simulink model "TST_OilP_DD"  (R2016b)
settings: Solver=FixedStepDiscrete  StartTime=0.0  StopTime=simTime  FixedStep=sampleTime  RelTol=1e-3
values from neighbouring files (symbols this model uses):
  testCase = 1    [initTST_OilP_DD_001.m]
libraries: simulink x13, UnitTest_Lib x11
settings Model: Creator=xinchangran  LastModifiedBy=xinchangran
settings DebuggingCC: SignalRangeChecking=error

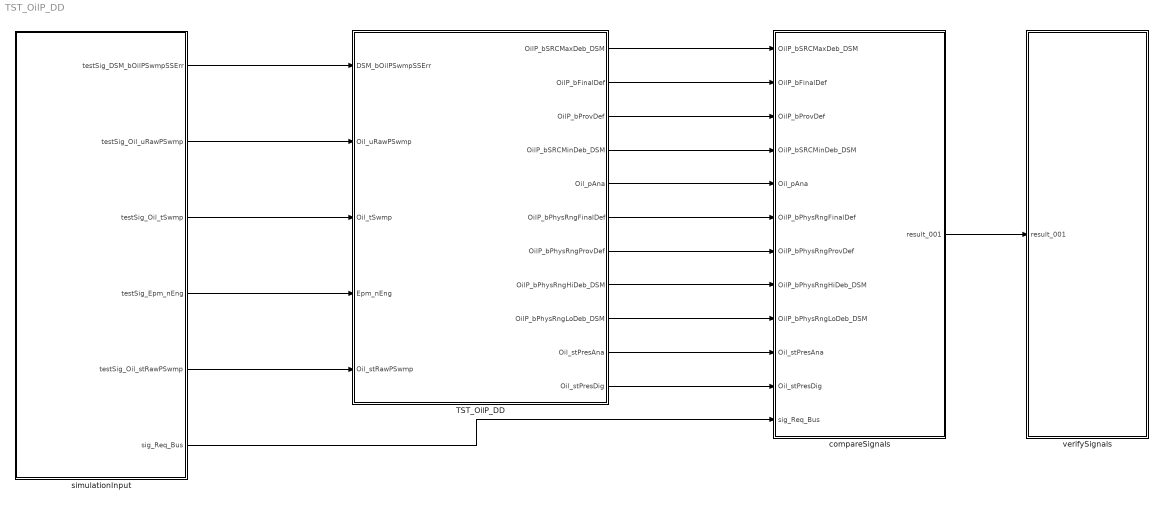
== system TST_OilP_DD ==
  TST_OilP_DD : Subsystem
  compareSignals : Subsystem
  simulationInput : Subsystem
  verifySignals : Subsystem
  wires:
  simulationInput/1(testSig_DSM_bOilPSwmpSSErr) -> TST_OilP_DD/1(DSM_bOilPSwmpSSErr)
  simulationInput/2(testSig_Oil_uRawPSwmp) -> TST_OilP_DD/2(Oil_uRawPSwmp)
  simulationInput/3(testSig_Oil_tSwmp) -> TST_OilP_DD/3(Oil_tSwmp)
  simulationInput/4(testSig_Epm_nEng) -> TST_OilP_DD/4(Epm_nEng)
  simulationInput/5(testSig_Oil_stRawPSwmp) -> TST_OilP_DD/5(Oil_stRawPSwmp)
  TST_OilP_DD/1(OilP_bSRCMaxDeb_DSM) -> compareSignals/1(OilP_bSRCMaxDeb_DSM)
  TST_OilP_DD/2(OilP_bFinalDef) -> compareSignals/2(OilP_bFinalDef)
  TST_OilP_DD/3(OilP_bProvDef) -> compareSignals/3(OilP_bProvDef)
  TST_OilP_DD/4(OilP_bSRCMinDeb_DSM) -> compareSignals/4(OilP_bSRCMinDeb_DSM)
  TST_OilP_DD/5(Oil_pAna) -> compareSignals/5(Oil_pAna)
  TST_OilP_DD/6(OilP_bPhysRngFinalDef) -> compareSignals/6(OilP_bPhysRngFinalDef)
  TST_OilP_DD/7(OilP_bPhysRngProvDef) -> compareSignals/7(OilP_bPhysRngProvDef)
  TST_OilP_DD/8(OilP_bPhysRngHiDeb_DSM) -> compareSignals/8(OilP_bPhysRngHiDeb_DSM)
  TST_OilP_DD/9(OilP_bPhysRngLoDeb_DSM) -> compareSignals/9(OilP_bPhysRngLoDeb_DSM)
  TST_OilP_DD/10(Oil_stPresAna) -> compareSignals/10(Oil_stPresAna)
  TST_OilP_DD/11(Oil_stPresDig) -> compareSignals/11(Oil_stPresDig)
  simulationInput/6(sig_Req_Bus) -> compareSignals/12(sig_Req_Bus)
  compareSignals/1(result_001) -> verifySignals/1(result_001)

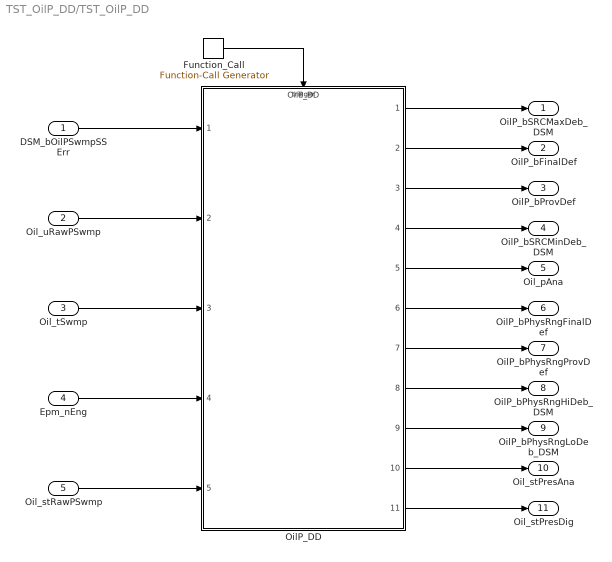
== system TST_OilP_DD/TST_OilP_DD ==
  DSM_bOilPSwmpSSErr : Inport
  Oil_uRawPSwmp : Inport  Port=2
  Oil_tSwmp : Inport  Port=3
  Epm_nEng : Inport  Port=4
  Oil_stRawPSwmp : Inport  Port=5
  Function_Call : simulink/Ports & Subsystems/Function-Call Generator  sample_time=sampleTime  numberOfIterations=1
  OilP_DD : ModelReference  ModelNameDialog=OilP_DD  SimulationMode=Normal  ModelReferenceVersion=1.40  TriggerPortName=function  TriggerPortTriggerType=function-call  TriggerPortStatesWhenEnabling=held
  OilP_bSRCMaxDeb_DSM : Outport
  OilP_bFinalDef : Outport  Port=2
  OilP_bProvDef : Outport  Port=3
  OilP_bSRCMinDeb_DSM : Outport  Port=4
  Oil_pAna : Outport  Port=5
  OilP_bPhysRngFinalDef : Outport  Port=6
  OilP_bPhysRngProvDef : Outport  Port=7
  OilP_bPhysRngHiDeb_DSM : Outport  Port=8
  OilP_bPhysRngLoDeb_DSM : Outport  Port=9
  Oil_stPresAna : Outport  Port=10
  Oil_stPresDig : Outport  Port=11
  wires:
  Function_Call/1 -> OilP_DD/Trigger
  DSM_bOilPSwmpSSErr/1 -> OilP_DD/1
  Oil_uRawPSwmp/1 -> OilP_DD/2
  Oil_tSwmp/1 -> OilP_DD/3
  Epm_nEng/1 -> OilP_DD/4
  Oil_stRawPSwmp/1 -> OilP_DD/5
  OilP_DD/1 -> OilP_bSRCMaxDeb_DSM/1
  OilP_DD/2 -> OilP_bFinalDef/1
  OilP_DD/3 -> OilP_bProvDef/1
  OilP_DD/4 -> OilP_bSRCMinDeb_DSM/1
  OilP_DD/5 -> Oil_pAna/1
  OilP_DD/6 -> OilP_bPhysRngFinalDef/1
  OilP_DD/7 -> OilP_bPhysRngProvDef/1
  OilP_DD/8 -> OilP_bPhysRngHiDeb_DSM/1
  OilP_DD/9 -> OilP_bPhysRngLoDeb_DSM/1
  OilP_DD/10 -> Oil_stPresAna/1
  OilP_DD/11 -> Oil_stPresDig/1

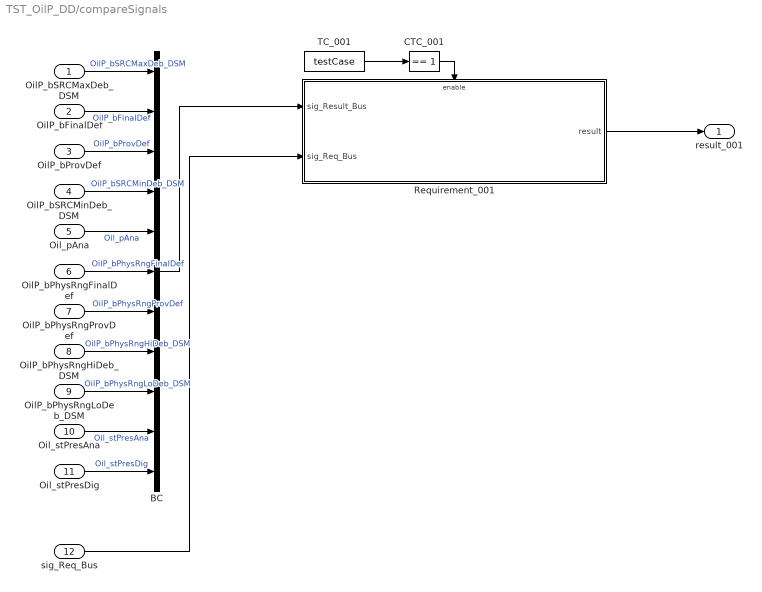
== system TST_OilP_DD/compareSignals ==
  OilP_bSRCMaxDeb_DSM : Inport
  OilP_bFinalDef : Inport  Port=2
  OilP_bProvDef : Inport  Port=3
  OilP_bSRCMinDeb_DSM : Inport  Port=4
  Oil_pAna : Inport  Port=5
  OilP_bPhysRngFinalDef : Inport  Port=6
  OilP_bPhysRngProvDef : Inport  Port=7
  OilP_bPhysRngHiDeb_DSM : Inport  Port=8
  OilP_bPhysRngLoDeb_DSM : Inport  Port=9
  Oil_stPresAna : Inport  Port=10
  Oil_stPresDig : Inport  Port=11
  sig_Req_Bus : Inport  Port=12
  BC : BusCreator  Inputs=11
  CTC_001 : simulink/Logic and Bit Operations/Compare To Constant  relop===  const=1  OutDataTypeStr=boolean
  Requirement_001 : Subsystem
  TC_001 : Constant  Value=testCase
  result_001 : Outport
  wires:
  OilP_bSRCMaxDeb_DSM/1 -> BC/1  "OilP_bSRCMaxDeb_DSM"
  OilP_bFinalDef/1 -> BC/2  "OilP_bFinalDef"
  OilP_bProvDef/1 -> BC/3  "OilP_bProvDef"
  OilP_bSRCMinDeb_DSM/1 -> BC/4  "OilP_bSRCMinDeb_DSM"
  Oil_pAna/1 -> BC/5  "Oil_pAna"
  OilP_bPhysRngFinalDef/1 -> BC/6  "OilP_bPhysRngFinalDef"
  OilP_bPhysRngProvDef/1 -> BC/7  "OilP_bPhysRngProvDef"
  OilP_bPhysRngHiDeb_DSM/1 -> BC/8  "OilP_bPhysRngHiDeb_DSM"
  OilP_bPhysRngLoDeb_DSM/1 -> BC/9  "OilP_bPhysRngLoDeb_DSM"
  Oil_stPresAna/1 -> BC/10  "Oil_stPresAna"
  Oil_stPresDig/1 -> BC/11  "Oil_stPresDig"
  TC_001/1 -> CTC_001/1
  CTC_001/1 -> Requirement_001/Enable
  sig_Req_Bus/1 -> Requirement_001/2(sig_Req_Bus)
  BC/1 -> Requirement_001/1(sig_Result_Bus)
  Requirement_001/1(result) -> result_001/1

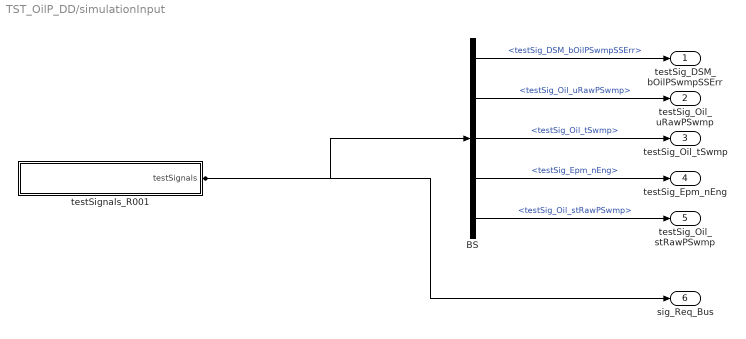
== system TST_OilP_DD/simulationInput ==
  BS : BusSelector  OutputSignals=testSig_DSM_bOilPSwmpSSErr,testSig_Oil_uRawPSwmp,testSig_Oil_tSwmp,testSig_Epm_nEng,testSig_Oil_stRawPSwmp
  testSignals_R001 : Subsystem
  testSig_DSM_bOilPSwmpSSErr : Outport
  testSig_Oil_uRawPSwmp : Outport  Port=2
  testSig_Oil_tSwmp : Outport  Port=3
  testSig_Epm_nEng : Outport  Port=4
  testSig_Oil_stRawPSwmp : Outport  Port=5
  sig_Req_Bus : Outport  Port=6
  wires:
  BS/1 -> testSig_DSM_bOilPSwmpSSErr/1  "<testSig_DSM_bOilPSwmpSSErr>"
  BS/2 -> testSig_Oil_uRawPSwmp/1  "<testSig_Oil_uRawPSwmp>"
  BS/3 -> testSig_Oil_tSwmp/1  "<testSig_Oil_tSwmp>"
  BS/4 -> testSig_Epm_nEng/1  "<testSig_Epm_nEng>"
  BS/5 -> testSig_Oil_stRawPSwmp/1  "<testSig_Oil_stRawPSwmp>"
  testSignals_R001/1(testSignals) -> BS/1, sig_Req_Bus/1

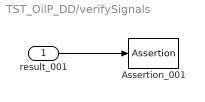
== system TST_OilP_DD/verifySignals ==
  result_001 : Inport
  Assertion_001 : Assertion  Enabled=off
  wires:
  result_001/1 -> Assertion_001/1

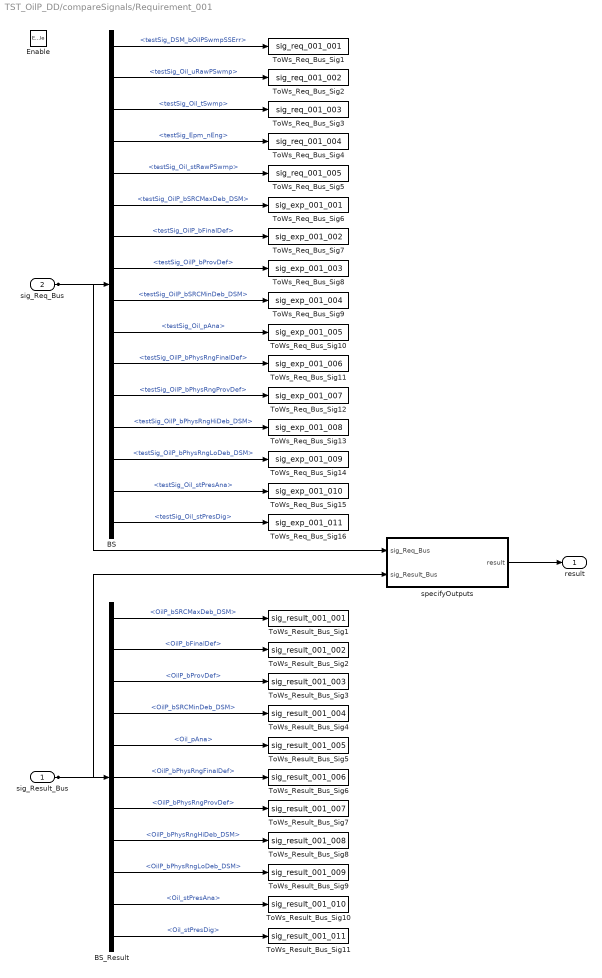
== system TST_OilP_DD/compareSignals/Requirement_001 ==
  sig_Result_Bus : Inport
  sig_Req_Bus : Inport  Port=2
  Enable : EnablePort
  BS : BusSelector  OutputSignals=testSig_DSM_bOilPSwmpSSErr,testSig_Oil_uRawPSwmp,testSig_Oil_tSwmp,testSig_Epm_nEng,testSig_Oil_stRawPSwmp,testSig_OilP_bSRCMaxDeb_DSM,testSig_OilP_bFinalDef,testSig_OilP_bProvDef,testSig_OilP_bSRCMinDeb_DSM,testSig_Oil_pAna,testSig_OilP_bPhysRngFinalDef,testSig_OilP_bPhysRngProvDef,testSig_OilP_bPhysRngHiDeb_DSM,testSig_OilP_bPhysRngLoDeb_DSM,testSig_Oil_stPresAna,testSig_Oil_stPresDig
  BS_Result : BusSelector  OutputSignals=OilP_bSRCMaxDeb_DSM,OilP_bFinalDef,OilP_bProvDef,OilP_bSRCMinDeb_DSM,Oil_pAna,OilP_bPhysRngFinalDef,OilP_bPhysRngProvDef,OilP_bPhysRngHiDeb_DSM,OilP_bPhysRngLoDeb_DSM,Oil_stPresAna,Oil_stPresDig
  ToWs_Req_Bus_Sig1 : ToWorkspace  VariableName=sig_req_001_001  SaveFormat=Structure With Time
  ToWs_Req_Bus_Sig10 : ToWorkspace  VariableName=sig_exp_001_005  SaveFormat=Structure With Time
  ToWs_Req_Bus_Sig11 : ToWorkspace  VariableName=sig_exp_001_006  SaveFormat=Structure With Time
  ToWs_Req_Bus_Sig12 : ToWorkspace  VariableName=sig_exp_001_007  SaveFormat=Structure With Time
  ToWs_Req_Bus_Sig13 : ToWorkspace  VariableName=sig_exp_001_008  SaveFormat=Structure With Time
  ToWs_Req_Bus_Sig14 : ToWorkspace  VariableName=sig_exp_001_009  SaveFormat=Structure With Time
  ToWs_Req_Bus_Sig15 : ToWorkspace  VariableName=sig_exp_001_010  SaveFormat=Structure With Time
  ToWs_Req_Bus_Sig16 : ToWorkspace  VariableName=sig_exp_001_011  SaveFormat=Structure With Time
  ToWs_Req_Bus_Sig2 : ToWorkspace  VariableName=sig_req_001_002  SaveFormat=Structure With Time
  ToWs_Req_Bus_Sig3 : ToWorkspace  VariableName=sig_req_001_003  SaveFormat=Structure With Time
  ToWs_Req_Bus_Sig4 : ToWorkspace  VariableName=sig_req_001_004  SaveFormat=Structure With Time
  ToWs_Req_Bus_Sig5 : ToWorkspace  VariableName=sig_req_001_005  SaveFormat=Structure With Time
  ToWs_Req_Bus_Sig6 : ToWorkspace  VariableName=sig_exp_001_001  SaveFormat=Structure With Time
  ToWs_Req_Bus_Sig7 : ToWorkspace  VariableName=sig_exp_001_002  SaveFormat=Structure With Time
  ToWs_Req_Bus_Sig8 : ToWorkspace  VariableName=sig_exp_001_003  SaveFormat=Structure With Time
  ToWs_Req_Bus_Sig9 : ToWorkspace  VariableName=sig_exp_001_004  SaveFormat=Structure With Time
  ToWs_Result_Bus_Sig1 : ToWorkspace  VariableName=sig_result_001_001  SaveFormat=Structure With Time
  ToWs_Result_Bus_Sig10 : ToWorkspace  VariableName=sig_result_001_010  SaveFormat=Structure With Time
  ToWs_Result_Bus_Sig11 : ToWorkspace  VariableName=sig_result_001_011  SaveFormat=Structure With Time
  ToWs_Result_Bus_Sig2 : ToWorkspace  VariableName=sig_result_001_002  SaveFormat=Structure With Time
  ToWs_Result_Bus_Sig3 : ToWorkspace  VariableName=sig_result_001_003  SaveFormat=Structure With Time
  ToWs_Result_Bus_Sig4 : ToWorkspace  VariableName=sig_result_001_004  SaveFormat=Structure With Time
  ToWs_Result_Bus_Sig5 : ToWorkspace  VariableName=sig_result_001_005  SaveFormat=Structure With Time
  ToWs_Result_Bus_Sig6 : ToWorkspace  VariableName=sig_result_001_006  SaveFormat=Structure With Time
  ToWs_Result_Bus_Sig7 : ToWorkspace  VariableName=sig_result_001_007  SaveFormat=Structure With Time
  ToWs_Result_Bus_Sig8 : ToWorkspace  VariableName=sig_result_001_008  SaveFormat=Structure With Time
  ToWs_Result_Bus_Sig9 : ToWorkspace  VariableName=sig_result_001_009  SaveFormat=Structure With Time
  specifyOutputs : Subsystem
  result : Outport
  wires:
  sig_Req_Bus/1 -> BS/1, specifyOutputs/1(sig_Req_Bus)
  BS/1 -> ToWs_Req_Bus_Sig1/1  "<testSig_DSM_bOilPSwmpSSErr>"
  BS/2 -> ToWs_Req_Bus_Sig2/1  "<testSig_Oil_uRawPSwmp>"
  BS/3 -> ToWs_Req_Bus_Sig3/1  "<testSig_Oil_tSwmp>"
  BS/4 -> ToWs_Req_Bus_Sig4/1  "<testSig_Epm_nEng>"
  BS/5 -> ToWs_Req_Bus_Sig5/1  "<testSig_Oil_stRawPSwmp>"
  BS/6 -> ToWs_Req_Bus_Sig6/1  "<testSig_OilP_bSRCMaxDeb_DSM>"
  BS/7 -> ToWs_Req_Bus_Sig7/1  "<testSig_OilP_bFinalDef>"
  BS/8 -> ToWs_Req_Bus_Sig8/1  "<testSig_OilP_bProvDef>"
  BS/9 -> ToWs_Req_Bus_Sig9/1  "<testSig_OilP_bSRCMinDeb_DSM>"
  BS/10 -> ToWs_Req_Bus_Sig10/1  "<testSig_Oil_pAna>"
  BS/11 -> ToWs_Req_Bus_Sig11/1  "<testSig_OilP_bPhysRngFinalDef>"
  BS/12 -> ToWs_Req_Bus_Sig12/1  "<testSig_OilP_bPhysRngProvDef>"
  BS/13 -> ToWs_Req_Bus_Sig13/1  "<testSig_OilP_bPhysRngHiDeb_DSM>"
  BS/14 -> ToWs_Req_Bus_Sig14/1  "<testSig_OilP_bPhysRngLoDeb_DSM>"
  BS/15 -> ToWs_Req_Bus_Sig15/1  "<testSig_Oil_stPresAna>"
  BS/16 -> ToWs_Req_Bus_Sig16/1  "<testSig_Oil_stPresDig>"
  sig_Result_Bus/1 -> BS_Result/1, specifyOutputs/2(sig_Result_Bus)
  BS_Result/1 -> ToWs_Result_Bus_Sig1/1  "<OilP_bSRCMaxDeb_DSM>"
  BS_Result/2 -> ToWs_Result_Bus_Sig2/1  "<OilP_bFinalDef>"
  BS_Result/3 -> ToWs_Result_Bus_Sig3/1  "<OilP_bProvDef>"
  BS_Result/4 -> ToWs_Result_Bus_Sig4/1  "<OilP_bSRCMinDeb_DSM>"
  BS_Result/5 -> ToWs_Result_Bus_Sig5/1  "<Oil_pAna>"
  BS_Result/6 -> ToWs_Result_Bus_Sig6/1  "<OilP_bPhysRngFinalDef>"
  BS_Result/7 -> ToWs_Result_Bus_Sig7/1  "<OilP_bPhysRngProvDef>"
  BS_Result/8 -> ToWs_Result_Bus_Sig8/1  "<OilP_bPhysRngHiDeb_DSM>"
  BS_Result/9 -> ToWs_Result_Bus_Sig9/1  "<OilP_bPhysRngLoDeb_DSM>"
  BS_Result/10 -> ToWs_Result_Bus_Sig10/1  "<Oil_stPresAna>"
  BS_Result/11 -> ToWs_Result_Bus_Sig11/1  "<Oil_stPresDig>"
  specifyOutputs/1(result) -> result/1

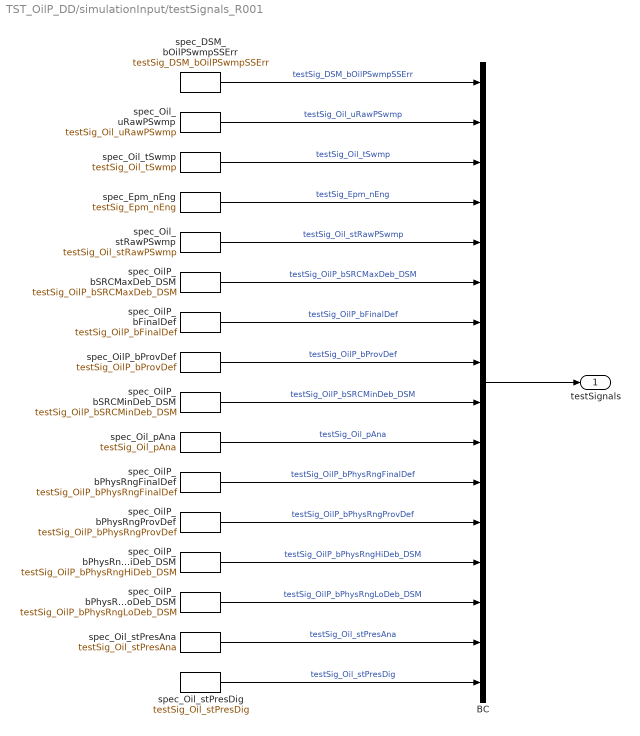
== system TST_OilP_DD/simulationInput/testSignals_R001 ==
  BC : BusCreator  Inputs=16
  spec_DSM_bOilPSwmpSSErr : FromWorkspace  VariableName=testSig_DSM_bOilPSwmpSSErr  Interpolate=off  OutputAfterFinalValue=Holding final value
  spec_Epm_nEng : FromWorkspace  VariableName=testSig_Epm_nEng  Interpolate=off  OutputAfterFinalValue=Holding final value
  spec_OilP_bFinalDef : FromWorkspace  VariableName=testSig_OilP_bFinalDef  Interpolate=off  OutputAfterFinalValue=Holding final value
  spec_OilP_bPhysRngFinalDef : FromWorkspace  VariableName=testSig_OilP_bPhysRngFinalDef  Interpolate=off  OutputAfterFinalValue=Holding final value
  spec_OilP_bPhysRngHiDeb_DSM : FromWorkspace  VariableName=testSig_OilP_bPhysRngHiDeb_DSM  Interpolate=off  OutputAfterFinalValue=Holding final value
  spec_OilP_bPhysRngLoDeb_DSM : FromWorkspace  VariableName=testSig_OilP_bPhysRngLoDeb_DSM  Interpolate=off  OutputAfterFinalValue=Holding final value
  spec_OilP_bPhysRngProvDef : FromWorkspace  VariableName=testSig_OilP_bPhysRngProvDef  Interpolate=off  OutputAfterFinalValue=Holding final value
  spec_OilP_bProvDef : FromWorkspace  VariableName=testSig_OilP_bProvDef  Interpolate=off  OutputAfterFinalValue=Holding final value
  spec_OilP_bSRCMaxDeb_DSM : FromWorkspace  VariableName=testSig_OilP_bSRCMaxDeb_DSM  Interpolate=off  OutputAfterFinalValue=Holding final value
  spec_OilP_bSRCMinDeb_DSM : FromWorkspace  VariableName=testSig_OilP_bSRCMinDeb_DSM  Interpolate=off  OutputAfterFinalValue=Holding final value
  spec_Oil_pAna : FromWorkspace  VariableName=testSig_Oil_pAna  Interpolate=off  OutputAfterFinalValue=Holding final value
  spec_Oil_stPresAna : FromWorkspace  VariableName=testSig_Oil_stPresAna  Interpolate=off  OutputAfterFinalValue=Holding final value
  spec_Oil_stPresDig : FromWorkspace  VariableName=testSig_Oil_stPresDig  Interpolate=off  OutputAfterFinalValue=Holding final value
  spec_Oil_stRawPSwmp : FromWorkspace  VariableName=testSig_Oil_stRawPSwmp  Interpolate=off  OutputAfterFinalValue=Holding final value
  spec_Oil_tSwmp : FromWorkspace  VariableName=testSig_Oil_tSwmp  Interpolate=off  OutputAfterFinalValue=Holding final value
  spec_Oil_uRawPSwmp : FromWorkspace  VariableName=testSig_Oil_uRawPSwmp  Interpolate=off  OutputAfterFinalValue=Holding final value
  testSignals : Outport
  wires:
  BC/1 -> testSignals/1
  spec_DSM_bOilPSwmpSSErr/1 -> BC/1  "testSig_DSM_bOilPSwmpSSErr"
  spec_Oil_uRawPSwmp/1 -> BC/2  "testSig_Oil_uRawPSwmp"
  spec_Oil_tSwmp/1 -> BC/3  "testSig_Oil_tSwmp"
  spec_Epm_nEng/1 -> BC/4  "testSig_Epm_nEng"
  spec_Oil_stRawPSwmp/1 -> BC/5  "testSig_Oil_stRawPSwmp"
  spec_OilP_bSRCMaxDeb_DSM/1 -> BC/6  "testSig_OilP_bSRCMaxDeb_DSM"
  spec_OilP_bFinalDef/1 -> BC/7  "testSig_OilP_bFinalDef"
  spec_OilP_bProvDef/1 -> BC/8  "testSig_OilP_bProvDef"
  spec_OilP_bSRCMinDeb_DSM/1 -> BC/9  "testSig_OilP_bSRCMinDeb_DSM"
  spec_Oil_pAna/1 -> BC/10  "testSig_Oil_pAna"
  spec_OilP_bPhysRngFinalDef/1 -> BC/11  "testSig_OilP_bPhysRngFinalDef"
  spec_OilP_bPhysRngProvDef/1 -> BC/12  "testSig_OilP_bPhysRngProvDef"
  spec_OilP_bPhysRngHiDeb_DSM/1 -> BC/13  "testSig_OilP_bPhysRngHiDeb_DSM"
  spec_OilP_bPhysRngLoDeb_DSM/1 -> BC/14  "testSig_OilP_bPhysRngLoDeb_DSM"
  spec_Oil_stPresAna/1 -> BC/15  "testSig_Oil_stPresAna"
  spec_Oil_stPresDig/1 -> BC/16  "testSig_Oil_stPresDig"

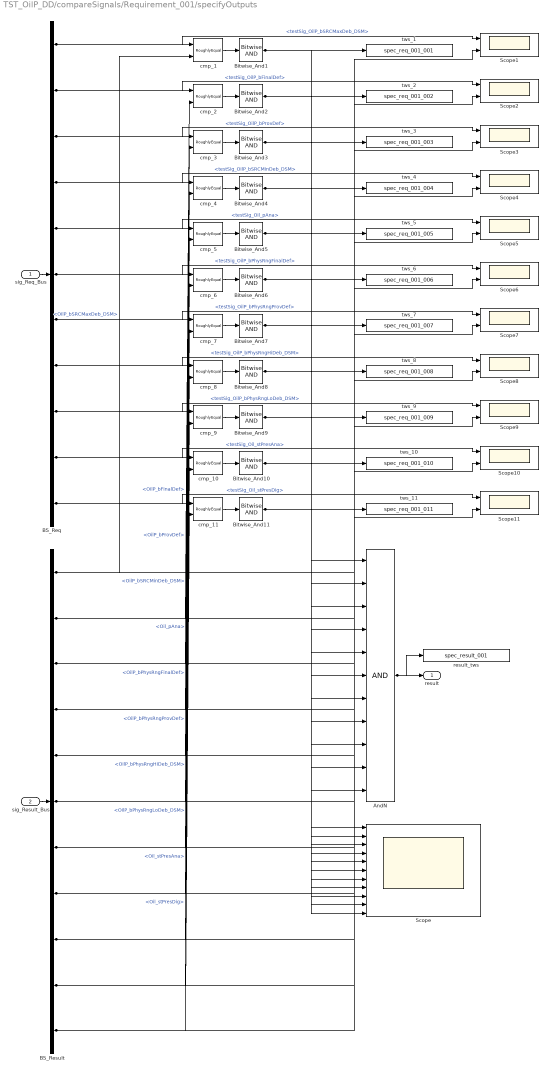
== system TST_OilP_DD/compareSignals/Requirement_001/specifyOutputs ==
  sig_Req_Bus : Inport
  sig_Result_Bus : Inport  Port=2
  AndN : Logic  Inputs=11
  BS_Req : BusSelector  OutputSignals=testSig_OilP_bSRCMaxDeb_DSM,testSig_OilP_bFinalDef,testSig_OilP_bProvDef,testSig_OilP_bSRCMinDeb_DSM,testSig_Oil_pAna,testSig_OilP_bPhysRngFinalDef,testSig_OilP_bPhysRngProvDef,testSig_OilP_bPhysRngHiDeb_DSM,testSig_OilP_bPhysRngLoDeb_DSM,testSig_Oil_stPresAna,testSig_Oil_stPresDig
  BS_Result : BusSelector  OutputSignals=OilP_bSRCMaxDeb_DSM,OilP_bFinalDef,OilP_bProvDef,OilP_bSRCMinDeb_DSM,Oil_pAna,OilP_bPhysRngFinalDef,OilP_bPhysRngProvDef,OilP_bPhysRngHiDeb_DSM,OilP_bPhysRngLoDeb_DSM,Oil_stPresAna,Oil_stPresDig
  Bitwise_And{1..11} (11 alike) : simulink/Logic and Bit Operations/Bitwise Operator  logicop=AND  UseBitMask=off  BitMask=bin2dec('11011001')  BitMaskRealWorld=Stored Integer
  Scope : Scope  NumInputPorts=11
  Scope{1..11} (11 alike) : Scope  NumInputPorts=2
  cmp_{1..11} (11 alike) : UnitTest_Lib/RoughlyEqual  slope=0.1
  result_tws : ToWorkspace  VariableName=spec_result_001
  tws_1 : ToWorkspace  VariableName=spec_req_001_001
  tws_10 : ToWorkspace  VariableName=spec_req_001_010
  tws_11 : ToWorkspace  VariableName=spec_req_001_011
  tws_2 : ToWorkspace  VariableName=spec_req_001_002
  tws_3 : ToWorkspace  VariableName=spec_req_001_003
  tws_4 : ToWorkspace  VariableName=spec_req_001_004
  tws_5 : ToWorkspace  VariableName=spec_req_001_005
  tws_6 : ToWorkspace  VariableName=spec_req_001_006
  tws_7 : ToWorkspace  VariableName=spec_req_001_007
  tws_8 : ToWorkspace  VariableName=spec_req_001_008
  tws_9 : ToWorkspace  VariableName=spec_req_001_009
  result : Outport
  wires:
  sig_Req_Bus/1 -> BS_Req/1
  sig_Result_Bus/1 -> BS_Result/1
  AndN/1 -> result/1, result_tws/1
  BS_Req/1 -> cmp_1/1, Scope1/1  "<testSig_OilP_bSRCMaxDeb_DSM>"
  BS_Result/1 -> cmp_1/2, Scope1/2  "<OilP_bSRCMaxDeb_DSM>"
  cmp_1/1 -> Bitwise_And1/1
  Bitwise_And1/1 -> tws_1/1, AndN/1, Scope/1
  BS_Req/2 -> cmp_2/1, Scope2/1  "<testSig_OilP_bFinalDef>"
  BS_Result/2 -> cmp_2/2, Scope2/2  "<OilP_bFinalDef>"
  cmp_2/1 -> Bitwise_And2/1
  Bitwise_And2/1 -> tws_2/1, AndN/2, Scope/2
  BS_Req/3 -> cmp_3/1, Scope3/1  "<testSig_OilP_bProvDef>"
  BS_Result/3 -> cmp_3/2, Scope3/2  "<OilP_bProvDef>"
  cmp_3/1 -> Bitwise_And3/1
  Bitwise_And3/1 -> tws_3/1, AndN/3, Scope/3
  BS_Req/4 -> cmp_4/1, Scope4/1  "<testSig_OilP_bSRCMinDeb_DSM>"
  BS_Result/4 -> cmp_4/2, Scope4/2  "<OilP_bSRCMinDeb_DSM>"
  cmp_4/1 -> Bitwise_And4/1
  Bitwise_And4/1 -> tws_4/1, AndN/4, Scope/4
  BS_Req/5 -> cmp_5/1, Scope5/1  "<testSig_Oil_pAna>"
  BS_Result/5 -> cmp_5/2, Scope5/2  "<Oil_pAna>"
  cmp_5/1 -> Bitwise_And5/1
  Bitwise_And5/1 -> tws_5/1, AndN/5, Scope/5
  BS_Req/6 -> cmp_6/1, Scope6/1  "<testSig_OilP_bPhysRngFinalDef>"
  BS_Result/6 -> cmp_6/2, Scope6/2  "<OilP_bPhysRngFinalDef>"
  cmp_6/1 -> Bitwise_And6/1
  Bitwise_And6/1 -> tws_6/1, AndN/6, Scope/6
  BS_Req/7 -> cmp_7/1, Scope7/1  "<testSig_OilP_bPhysRngProvDef>"
  BS_Result/7 -> cmp_7/2, Scope7/2  "<OilP_bPhysRngProvDef>"
  cmp_7/1 -> Bitwise_And7/1
  Bitwise_And7/1 -> tws_7/1, AndN/7, Scope/7
  BS_Req/8 -> cmp_8/1, Scope8/1  "<testSig_OilP_bPhysRngHiDeb_DSM>"
  BS_Result/8 -> cmp_8/2, Scope8/2  "<OilP_bPhysRngHiDeb_DSM>"
  cmp_8/1 -> Bitwise_And8/1
  Bitwise_And8/1 -> tws_8/1, AndN/8, Scope/8
  BS_Req/9 -> cmp_9/1, Scope9/1  "<testSig_OilP_bPhysRngLoDeb_DSM>"
  BS_Result/9 -> cmp_9/2, Scope9/2  "<OilP_bPhysRngLoDeb_DSM>"
  cmp_9/1 -> Bitwise_And9/1
  Bitwise_And9/1 -> tws_9/1, AndN/9, Scope/9
  BS_Req/10 -> cmp_10/1, Scope10/1  "<testSig_Oil_stPresAna>"
  BS_Result/10 -> cmp_10/2, Scope10/2  "<Oil_stPresAna>"
  cmp_10/1 -> Bitwise_And10/1
  Bitwise_And10/1 -> tws_10/1, AndN/10, Scope/10
  BS_Req/11 -> cmp_11/1, Scope11/1  "<testSig_Oil_stPresDig>"
  BS_Result/11 -> cmp_11/2, Scope11/2  "<Oil_stPresDig>"
  cmp_11/1 -> Bitwise_And11/1
  Bitwise_And11/1 -> tws_11/1, AndN/11, Scope/11
